simulink subsystem "HEVP1SSC"  (R2025b)
settings: Solver=VariableStepAuto  StartTime=0.0  StopTime=10.0  RelTol=1e-3
undefined symbols (not defined in the file): PlntEM1RotInertia, PlntEngInertia
libraries: fl_lib x1
settings Model: ModifiedByFormat=The MathWorks, Inc.  Creator=The MathWorks, Inc.  LastModifiedBy=The MathWorks, Inc.
settings OptimizationCC: ReuseModelBlockBuffer=off
settings RTWCC: GPUComputeCapability=3.5

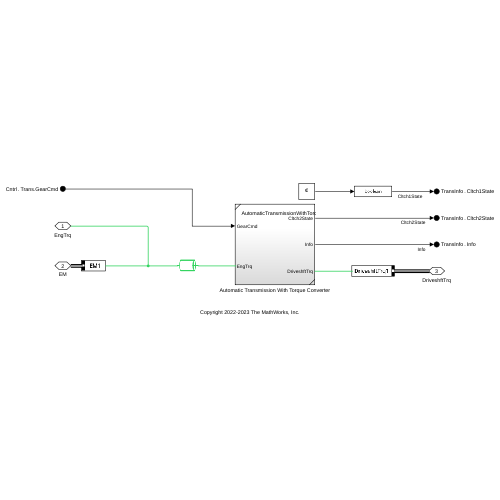
[thumbnail: Simulink's stored preview of the top-level diagram]
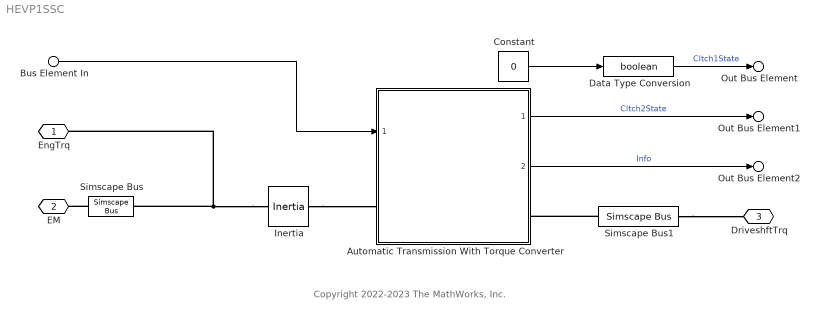
== system HEVP1SSC ==
  note: Copyright 2022-2023 The MathWorks, Inc.
  Bus Element In : Inport  PortName=Cntrl  Element=Trans.GearCmd
  Automatic Transmission With Torque Converter : Subsystem  ReferencedSubsystem=AutomaticTransmissionWithTorqueConverterSSC
  Constant : Constant  Value=0  SampleTime=-1
  Data Type Conversion : DataTypeConversion  OutDataTypeStr=boolean  SaturateOnIntegerOverflow=off  RndMeth=Floor
  Inertia : fl_lib/Mechanical/Rotational Elements/Inertia  inertia=PlntEngInertia + PlntEM1RotInertia kg*m^2  num_ports=foundation.enum.numPorts2.two  w_specify=off  w_priority=High  w=0 rad/s  w_nominal_specify=off  w_nominal_value=1  w_nominal_unit=rad/s  t_specify=off  t_priority=None  t=0 N*m  t_nominal_specify=off  t_nominal_value=1  t_nominal_unit=N*m
      settings: InternalSimscapePortConfiguration="{\"Bottom\":[],\"Left\":[{\"id\":\"I\",\"label\":\"\",\"type\":\"foundation.mechanical.rotational.rotational\"}],\"Right\":[{\"id\":\"J\",\"label\":\"\",\"type\":\"foundation.mechanical.rotational.rotational\"}],\"Top\":[]}"
  Simscape Bus : SimscapeBus  HierarchyStrings=EM1
  Simscape Bus1 : SimscapeBus  HierarchyStrings=DriveshftTrq1
  EngTrq : PMIOPort  Side=Left
  EM : PMIOPort  Port=2  Side=Left
  DriveshftTrq : PMIOPort  Port=3  Side=Right
  Out Bus Element : Outport  PortName=TransInfo  Element=Cltch1State
  Out Bus Element1 : Outport  PortName=TransInfo  Element=Cltch2State
  Out Bus Element2 : Outport  PortName=TransInfo  Element=Info
  wires:
  Constant/1 -> Data Type Conversion/1
  Automatic Transmission With Torque Converter/2 -> Out Bus Element2/1  "Info"
  Automatic Transmission With Torque Converter/1 -> Out Bus Element1/1  "Cltch2State"
  Bus Element In/1 -> Automatic Transmission With Torque Converter/1
  Data Type Conversion/1 -> Out Bus Element/1  "Cltch1State"
  connections:
  Inertia/LConn1 -- Automatic Transmission With Torque Converter/LConn1
  Inertia/RConn1 -- EngTrq/RConn1 -- Simscape Bus/LConn1
  Simscape Bus/RConn1 -- EM/RConn1
  Simscape Bus1/RConn1 -- DriveshftTrq/RConn1
  Simscape Bus1/LConn1 -- Automatic Transmission With Torque Converter/RConn1
